simulink model "trim_model_lab_1"  (R2021b)
settings: Solver=VariableStepAuto  StartTime=0.0  StopTime=10.0  RelTol=1e-3
values from neighbouring files (symbols this model uses):
  a11 = -3    [script_lab_1.m]
  a12 = -2    [script_lab_1.m]
  a21 = -5    [script_lab_1.m]
  a22 = -6    [script_lab_1.m]
  b11 = 3    [script_lab_1.m]
  b12 = 7    [script_lab_1.m]
settings Model: Creator=79159  LastModifiedBy=79159

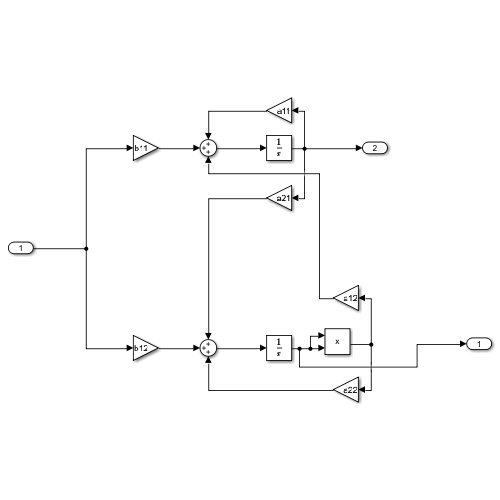
[thumbnail: Simulink's stored preview of the top-level diagram]
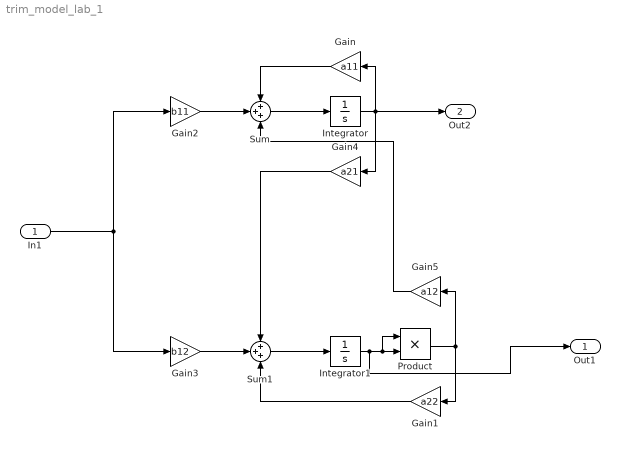
== system trim_model_lab_1 ==
  In1 : Inport
  Gain : Gain  Gain=a11
  Gain1 : Gain  Gain=a22
  Gain2 : Gain  Gain=b11
  Gain3 : Gain  Gain=b12
  Gain4 : Gain  Gain=a21
  Gain5 : Gain  Gain=a12
  Integrator : Integrator
  Integrator1 : Integrator
  Product : Product
  Sum : Sum  Inputs=+++
  Sum1 : Sum  Inputs=+++
  Out1 : Outport
  Out2 : Outport  Port=2
  wires:
  Gain1/1 -> Sum1/3
  In1/1 -> Gain2/1, Gain3/1
  Gain3/1 -> Sum1/2
  Gain2/1 -> Sum/2
  Product/1 -> Gain5/1, Gain1/1
  Gain4/1 -> Sum1/1
  Gain/1 -> Sum/1
  Sum/1 -> Integrator/1
  Integrator1/1 -> Out1/1, Product/1, Product/2
  Sum1/1 -> Integrator1/1
  Integrator/1 -> Out2/1, Gain/1, Gain4/1
  Gain5/1 -> Sum/3
